simulink model "skillwithfilterdoubletuned"  (R2017a)
settings: Solver=VariableStepAuto  StartTime=0.0  StopTime=10.0  MaxStep=1e-4  RelTol=1e-3
libraries: powerlib x20
settings Model: Creator=sakth  LastModifiedBy=sakth

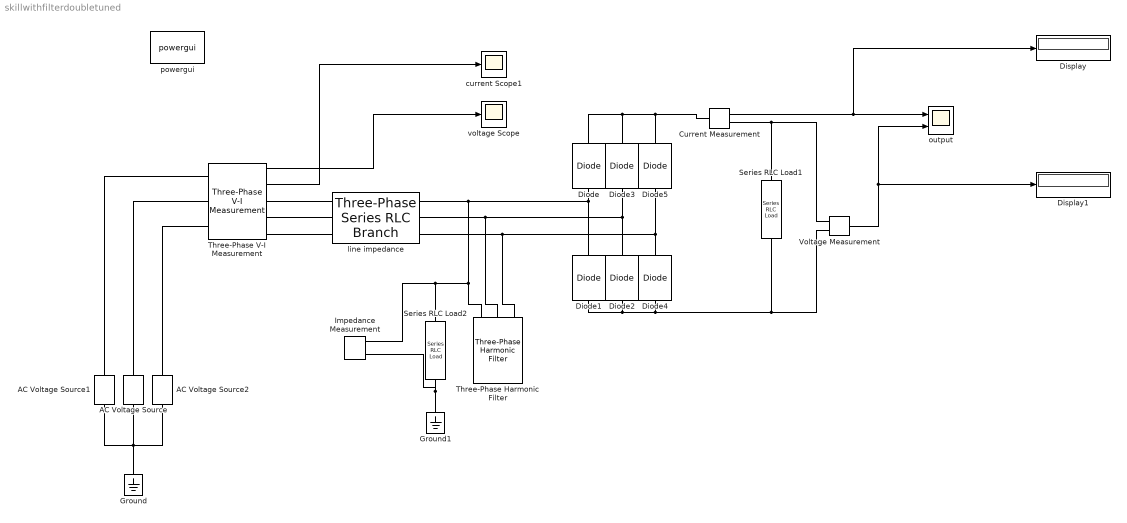
== system skillwithfilterdoubletuned ==
  AC Voltage Source : powerlib/Electrical Sources/AC Voltage Source  Amplitude=215  Phase=240  Frequency=50  SampleTime=0  Measurements=None  BusType=swing  Pref=10e3  Qref=0  Qmin=-inf  Qmax=+inf
  AC Voltage Source1 : powerlib/Electrical Sources/AC Voltage Source  Amplitude=215  Phase=120  Frequency=50  SampleTime=0  Measurements=None  BusType=swing  Pref=10e3  Qref=0  Qmin=-inf  Qmax=+inf
  AC Voltage Source2 : powerlib/Electrical Sources/AC Voltage Source  Amplitude=215  Phase=360  Frequency=50  SampleTime=0  Measurements=None  BusType=swing  Pref=10e3  Qref=0  Qmin=-inf  Qmax=+inf
  Current Measurement : powerlib/Measurements/Current Measurement  PhasorSimulation=off  OutputType=Complex  PSBequivalent=0
  Diode{,1..5} (6 alike) : powerlib/Power Electronics/Diode  Ron=0.001  Lon=0  Vf=0.8  IC=0  UseSnubber=off  Rs=500  Cs=250e-9  Measurements=off
  Display : Display
  Display1 : Display
  Ground : powerlib/Elements/Ground  LConnTagsString=a
  Ground1 : powerlib/Elements/Ground  LConnTagsString=a
  Impedance Measurement : powerlib/Measurements/Impedance Measurement  LConnTagsString=+|-  Factor=1
      settings: SourceProductName=Simscape Power Systems  SourceProductBaseCode=PS
  Series RLC Load1 : powerlib/Elements/Series RLC Load  LConnTagsString=a  RConnTagsString=__new0  NominalVoltage=1000  NominalFrequency=50  ActivePower=10e3  InductivePower=100  CapacitivePower=0  Setx0=off  InitialVoltage=0  SetiL0=off  InitialCurrent=0  Measurements=None  LoadType=constant Z
  Series RLC Load2 : powerlib/Elements/Series RLC Load  LConnTagsString=a  RConnTagsString=__new0  NominalVoltage=1000  NominalFrequency=50  ActivePower=10e3  InductivePower=0  CapacitivePower=0  Setx0=off  InitialVoltage=0  SetiL0=off  InitialCurrent=0  Measurements=None  LoadType=constant Z
  Three-Phase Harmonic Filter : powerlib/Elements/Three-Phase Harmonic Filter  LConnTagsString=A|B|C  FilterType=Double-tuned  FilterConnection=Y (grounded)  ParNom=[33e3 50]  Qc=6.2e6  Fr=[5*50]  Frd=[11*60 13*60]  Q=60  Measurements=None
      settings: AttributesFormatString=\n  SourceProductName=Simscape Power Systems  SourceProductBaseCode=PS
  Three-Phase V-I Measurement : powerlib/Measurements/Three-Phase V-I Measurement  VoltageMeasurement=phase-to-ground  SetLabelV=off  LabelV=Vabc  Vpu=off  VpuLL=off  CurrentMeasurement=yes  SetLabelI=off  LabelI=Iabc  Ipu=off  Pbase=100e6  Vbase=500e3  OutputType=Complex  PhasorSimulation=off  PSBequivalent=0
  Voltage Measurement : powerlib/Measurements/Voltage Measurement  PhasorSimulation=off  OutputType=Complex  PSBequivalent=0
  current Scope1 : Scope
  line impedance : powerlib/Elements/Three-Phase Series RLC Branch  LConnTagsString=A|B|C  RConnTagsString=A|B|C  BranchType=RL  Resistance=1  Inductance=0.1e-3  Capacitance=1e-6  Measurements=None
  output : Scope  NumInputPorts=2
  powergui : powerlib/powergui  Priority=1  SimulationMode=Continuous  SampleTime=50e-6  frequency=60  Iterations=50  frequencyindice=50  Pbase=100e6  ErrMax=1e-4  UnitsV=kV  UnitsW=MW  buscounter=0  FunctionMessages=off  echomessages=off  EnableUseOfTLC=off  CurrentSourceSwitches=off  DisableSnubberDevices=off  DisableRonSwitches=off  DisableVfSwitches=off  DisplayEquations=off  SolverType=Tustin/Backward Euler (TBE)  Interpol=off  ExternalGateDelay=off  methode=off  Ts=100  x0status=blocks  SPID=on  SwTol=0  HookPort=off  RestoreLinks=warning  ResistiveCurrentMeasurement=off  Frange=[0:2:1000]  Ylog=off  Xlog=off  ShowGrid=off  save=off  variable=ZData  structure=ct  ZoomFFT=on  StartTime=9.8  cycles=10  DisplayStyle=1  fundamental=50  FreqAxis=off  MaxFrequency=1000  frequencyindicesteady=1  RmsSteady=1  display=off
  voltage Scope : Scope
  wires:
  Voltage Measurement/1 -> output/2, Display1/1
  Three-Phase V-I Measurement/2 -> current Scope1/1
  Current Measurement/1 -> output/1, Display/1
  Three-Phase V-I Measurement/1 -> voltage Scope/1
  connections:
  Diode1/RConn1 -- Diode/LConn1 -- line impedance/RConn1 -- Three-Phase Harmonic Filter/LConn1 -- Impedance Measurement/LConn1 -- Series RLC Load2/LConn1
  Ground/LConn1 -- AC Voltage Source2/LConn1 -- AC Voltage Source1/LConn1 -- AC Voltage Source/LConn1
  Diode5/RConn1 -- Current Measurement/LConn1 -- Diode3/RConn1 -- Diode/RConn1
  Diode4/RConn1 -- Diode5/LConn1 -- Three-Phase Harmonic Filter/LConn3 -- line impedance/RConn3
  Diode2/RConn1 -- Three-Phase Harmonic Filter/LConn2 -- line impedance/RConn2 -- Diode3/LConn1
  Diode4/LConn1 -- Voltage Measurement/LConn2 -- Series RLC Load1/RConn1 -- Diode1/LConn1 -- Diode2/LConn1
  Series RLC Load1/LConn1 -- Voltage Measurement/LConn1 -- Current Measurement/RConn1
  Series RLC Load2/RConn1 -- Impedance Measurement/LConn2 -- Ground1/LConn1
  Three-Phase V-I Measurement/LConn3 -- AC Voltage Source2/RConn1
  Three-Phase V-I Measurement/RConn3 -- line impedance/LConn3
  Three-Phase V-I Measurement/LConn1 -- AC Voltage Source1/RConn1
  Three-Phase V-I Measurement/RConn1 -- line impedance/LConn1
  Three-Phase V-I Measurement/LConn2 -- AC Voltage Source/RConn1
  Three-Phase V-I Measurement/RConn2 -- line impedance/LConn2
